simulink model "CircuitoRC2"  (R2020b)
settings: Solver=ode45  StartTime=0.0  StopTime=10.0  FixedStep=0.01  MaxStep=0.1  RelTol=1e-3
settings Model: Creator=Stefano  LastModifiedBy=Stefano

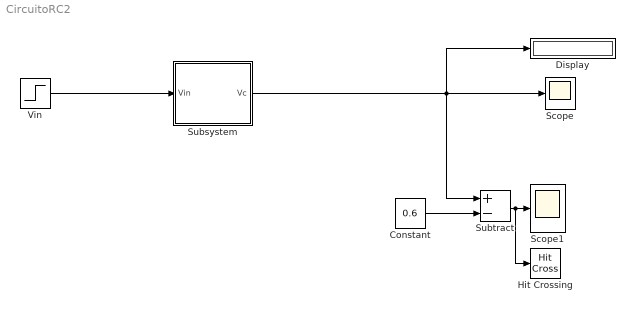
== system CircuitoRC2 ==
  Constant : Constant  Value=0.6
  Display : Display
  Hit Crossing : HitCross
  Scope : Scope
  Scope1 : Scope
  Subsystem : Subsystem  mask{par1=20, par2=0.1}
      mask prompts: par1 "R"; par2 "C"
      mask Display:
      | disp('RC circuit')
      | t=[0:0.1:10];
      | plot(t,1-exp(-t))
  Subtract : Sum  Inputs=+-
  Vin : Step  Time=2  SampleTime=0
  wires:
  Constant/1 -> Subtract/2
  Subtract/1 -> Hit Crossing/1, Scope1/1
  Subsystem/1(Vc) -> Display/1, Scope/1, Subtract/1
  Vin/1 -> Subsystem/1(Vin)

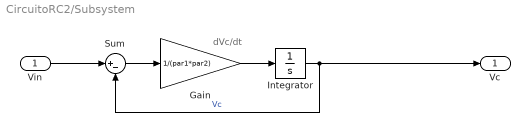
== system CircuitoRC2/Subsystem ==
  note: dVc/dt
  Vin : Inport
  Gain : Gain  Gain=1/(par1*par2)
  Integrator : Integrator
  Sum : Sum  Inputs=|+-
  Vc : Outport
  wires:
  Vin/1 -> Sum/1
  Integrator/1 -> Vc/1, Sum/2  "Vc"
  Sum/1 -> Gain/1
  Gain/1 -> Integrator/1
